simulink model "GainScheduledPIDBrakingSystem"  (Simulink 8.5)
settings: Solver=ode45  StartTime=0.0  StopTime=20  RelTol=1e-3
values from neighbouring files (symbols this model uses):
  C = xdotf:10:xdot0    [GainScheduledPIDTuner.m]
  Controllers = pidtune(Plants,'pidf',10)    [GainScheduledPIDTuner.m]
  distanceSet = x(n2:end)    [Trajectory.m]    (also in brakingTrajectory.m = [])
  P = 6894.76*Ppsi    (= 2757.904)    [allthesimulations.m]    (also in simParameters.m = 861.845)
  velocitySet = xdot(n2:end)    [Trajectory.m]    (also in brakingTrajectory.m = [])
undefined symbols (not defined in the file or in its folder): D, I, N
libraries: simulink x1
settings Model: Creator=MrPiccolo  LastModifiedBy=MrPiccolo
settings DataIOCC: SignalLoggingSaveFormat=Dataset
settings OptimizationCC: ExpressionDepthLimit=128
settings DebuggingCC: UnderspecifiedInitializationDetection=Simplified  MergeDetectMultiDrivingBlocksExec=error  FcnCallInpInsideContextMsg=EnableAllAsError  StateNameClashWarn=none
settings GRTTargetCC: CombineOutputUpdateFcns=on  GRTInterface=off

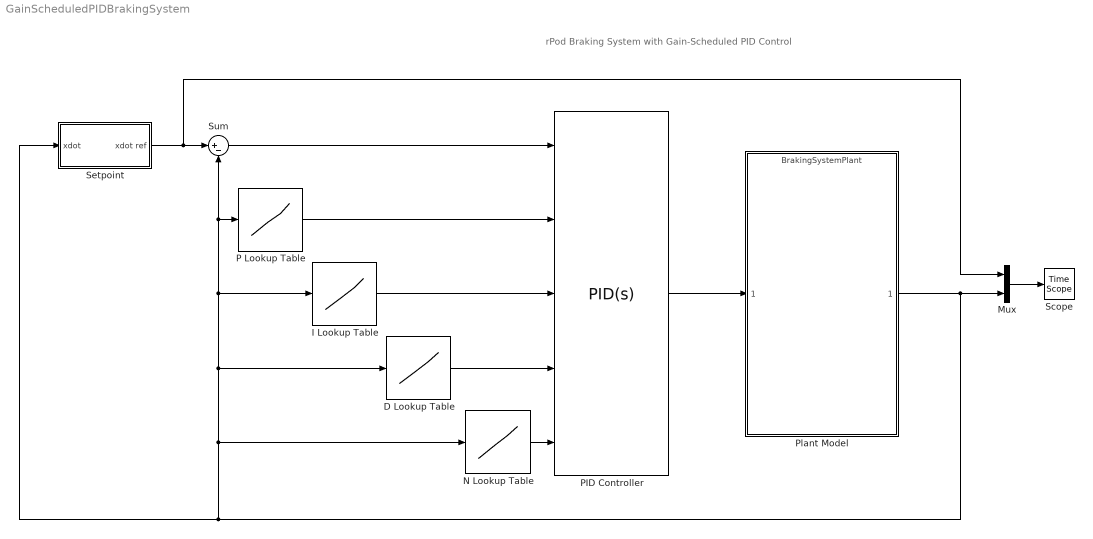
== system GainScheduledPIDBrakingSystem ==
  note: rPod Braking System
      | with Gain-Scheduled PID Control
  D Lookup Table : Lookup_n-D  NumberOfTableDimensions=1  BreakpointsForDimension1=C  Table=Controllers.Kd  ExtrapMethod=Clip  UseLastTableValue=on  InternalRulePriority=Speed  RndMeth=Simplest  InputSameDT=on
  I Lookup Table : Lookup_n-D  NumberOfTableDimensions=1  BreakpointsForDimension1=C  Table=Controllers.Ki  ExtrapMethod=Clip  UseLastTableValue=on  InternalRulePriority=Speed  RndMeth=Simplest  InputSameDT=on
  Mux : Mux  Inputs=2
  N Lookup Table : Lookup_n-D  NumberOfTableDimensions=1  BreakpointsForDimension1=C  Table=1./(Controllers.Tf)  ExtrapMethod=Clip  UseLastTableValue=on  InternalRulePriority=Speed  RndMeth=Simplest  InputSameDT=on
  P Lookup Table : Lookup_n-D  NumberOfTableDimensions=1  BreakpointsForDimension1=C  Table=Controllers.Kp  ExtrapMethod=Clip  UseLastTableValue=on  InternalRulePriority=Speed  RndMeth=Simplest  InputSameDT=on
  PID Controller : simulink/Continuous/PID Controller  Controller=PID  TimeDomain=Continuous-time  SampleTime=-1  IntegratorMethod=Forward Euler  FilterMethod=Forward Euler  Form=Parallel  UseFilter=on  ControllerParametersSource=external  P=P(1)  I=I(1)  D=D(1)  N=N(1)  InitialConditionSource=internal  InitialConditionForIntegrator=0  InitialConditionForFilter=0  ExternalReset=none  LimitOutput=off  UpperSaturationLimit=350  LowerSaturationLimit=250  LinearizeAsGain=on  AntiWindupMode=none  Kb=1  TrackingMode=off  Kt=1  PParamMin=[]  PParamMax=[]  IParamMin=[]  IParamMax=[]  DParamMin=[]  DParamMax=[]  NParamMin=[]  NParamMax=[]  KbParamMin=[]  KbParamMax=[]  KtParamMin=[]  KtParamMax=[]  POutMin=[]  POutMax=[]  IOutMin=[]  IOutMax=[]  DOutMin=[]  DOutMax=[]  NOutMin=[]  NOutMax=[]  KbOutMin=[]  KbOutMax=[]  KtOutMin=[]  KtOutMax=[]  IntegratorOutMin=[]  IntegratorOutMax=[]  FilterOutMin=[]  FilterOutMax=[]  SumOutMin=[]  SumOutMax=[]  SumI1OutMin=[]  SumI1OutMax=[]  SumI2OutMin=[]  SumI2OutMax=[]  SumI3OutMin=[]  SumI3OutMax=[]  SumDOutMin=[]  SumDOutMax=[]  SaturationOutMin=[]  SaturationOutMax=[]  IntegratorContinuousStateAttributes=''  IntegratorStateMustResolveToSignalObject=off  IntegratorRTWStateStorageClass=Auto  FilterContinuousStateAttributes=''  FilterStateMustResolveToSignalObject=off  FilterRTWStateStorageClass=Auto  DifferentiatorICPrevScaledInput=0  DifferentiatorOutMin=[]  DifferentiatorOutMax=[]
  Plant Model : ModelReference  ModelNameDialog=BrakingSystemPlant.mdl  SimulationMode=Normal  ModelReferenceVersion=1.147  CopyOfModelName=BrakingSystemPlant.mdl  DefaultDataLogging=on
  Scope : TimeScope
  Setpoint : Subsystem
  Sum : Sum  Inputs=|+-
  wires:
  Sum/1 -> PID Controller/1
  P Lookup Table/1 -> PID Controller/2
  I Lookup Table/1 -> PID Controller/3
  D Lookup Table/1 -> PID Controller/4
  N Lookup Table/1 -> PID Controller/5
  Setpoint/1(xdot ref) -> Mux/1, Sum/1
  Mux/1 -> Scope/1
  PID Controller/1 -> Plant Model/1
  Plant Model/1 -> Mux/2, Setpoint/1(xdot), Sum/2, P Lookup Table/1, I Lookup Table/1, D Lookup Table/1, N Lookup Table/1

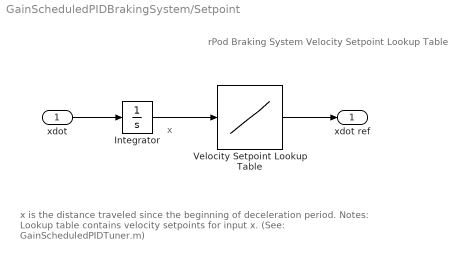
== system GainScheduledPIDBrakingSystem/Setpoint ==
  note: x is the distance traveled since the beginning of deceleration period.
      |
      | Notes:
      | Lookup table contains velocity setpoints for input x.
      | (See: GainScheduledPIDTuner.m)
  note: x
  note: rPod Braking System
      | Velocity Setpoint Lookup Table
  xdot : Inport
  Integrator : Integrator
  Velocity Setpoint Lookup Table : Lookup_n-D  NumberOfTableDimensions=1  BreakpointsForDimension1=distanceSet  Table=velocitySet  InternalRulePriority=Speed  RndMeth=Simplest  InputSameDT=on
  xdot ref : Outport
  wires:
  xdot/1 -> Integrator/1
  Integrator/1 -> Velocity Setpoint Lookup Table/1
  Velocity Setpoint Lookup Table/1 -> xdot ref/1
